simulink model "steamjacket"  (R2017b)
settings: Solver=VariableStepAuto  StartTime=0.0  StopTime=1000.0  RelTol=1e-3
settings Model: Creator=Bailey Brookes  LastModifiedBy=Bailey Brookes

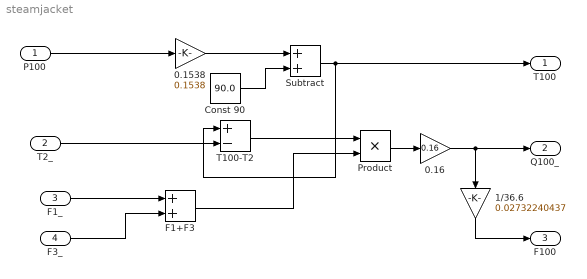
== system steamjacket ==
  P100 : Inport
  T2_ : Inport  Port=2
  F1_ : Inport  Port=3
  F3_ : Inport  Port=4
  0.1538 : Gain  Gain=0.1538
  0.16 : Gain  Gain=0.16
  1/36.6 : Gain  Gain=0.02732240437
  Const 90 : Constant  Value=90.0
  F1+F3 : Sum
  Product : Product
  Subtract : Sum
  T100-T2 : Sum  Inputs=+-
  T100 : Outport
  Q100_ : Outport  Port=2
  F100 : Outport  Port=3
  wires:
  F1+F3/1 -> Product/2
  Product/1 -> 0.16/1
  T2_/1 -> T100-T2/2
  T100-T2/1 -> Product/1
  Subtract/1 -> T100-T2/1, T100/1
  0.1538/1 -> Subtract/1
  F3_/1 -> F1+F3/2
  1/36.6/1 -> F100/1
  P100/1 -> 0.1538/1
  F1_/1 -> F1+F3/1
  Const 90/1 -> Subtract/2
  0.16/1 -> 1/36.6/1, Q100_/1
